simulink model "SVF_fromWorkspace"  (R2018b)
settings: Solver=VariableStepAuto  StartTime=0.0  StopTime=40  RelTol=1e-3
values from neighbouring files (symbols this model uses):
  a0 = omega_n^3    (= 31006276.6803)    [Tflex_Controller_init.m]
  a1 = 3*omega_n^2    (= 296088.132033)    [Tflex_Controller_init.m]
  a2 = 3*omega_n    (= 942.477796077)    [Tflex_Controller_init.m]
  svf_delay = round(svf_delay/(ts*10))    [Tflex_Controller_init.m]
  ts = 1/1000    (= 0.001)    [Tflex_Controller_init.m]
undefined symbols (not defined in the file or in its folder): DiscIntNeverNeededParam
settings Model: Creator=wout7  LastModifiedBy=wout7

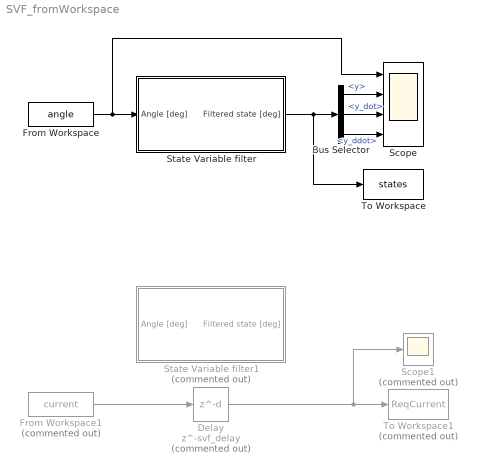
== system SVF_fromWorkspace ==
  Bus Selector : BusSelector  OutputSignals=y,y_dot,y_ddot
  Delay : Delay  Commented=on  DelayLength=svf_delay  SampleTime=ts
  From Workspace : FromWorkspace  VariableName=angle  SampleTime=ts
  From Workspace1 : FromWorkspace  Commented=on  VariableName=current  SampleTime=ts
  Scope : Scope  NumInputPorts=4
  Scope1 : Scope  Commented=on
  State Variable filter : Subsystem
  State Variable filter1 : Subsystem  Commented=on
  To Workspace : ToWorkspace  VariableName=states  SaveFormat=Timeseries  SampleTime=ts
  To Workspace1 : ToWorkspace  Commented=on  VariableName=ReqCurrent  SaveFormat=Timeseries  SampleTime=ts
  wires:
  From Workspace/1 -> Scope/1, State Variable filter/1(Angle [deg])
  State Variable filter/1(Filtered state [deg]) -> To Workspace/1, Bus Selector/1
  Bus Selector/2 -> Scope/3  "<y_dot>"
  Bus Selector/1 -> Scope/2  "<y>"
  Bus Selector/3 -> Scope/4  "<y_ddot>"
  From Workspace1/1 -> Delay/1
  Delay/1 -> Scope1/1, To Workspace1/1

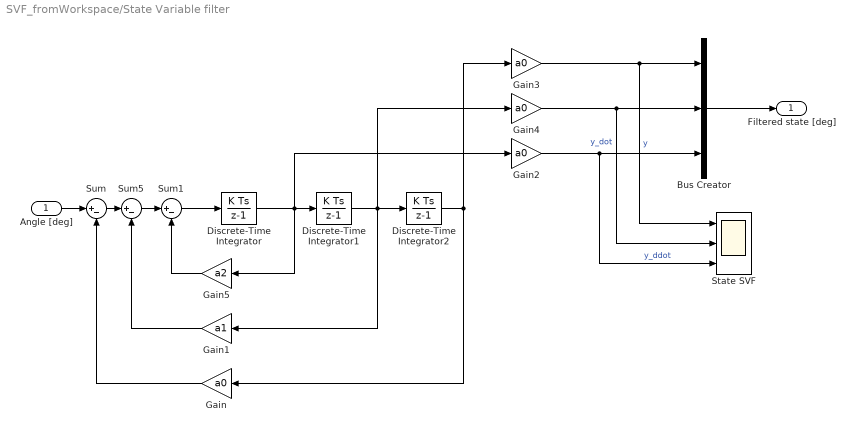
== system SVF_fromWorkspace/State Variable filter ==
  Angle [deg] : Inport
  Bus Creator : BusCreator  Inputs=3
  Discrete-Time Integrator : DiscreteIntegrator  SampleTime=-1  ICPrevOutput=DiscIntNeverNeededParam  ICPrevScaledInput=DiscIntNeverNeededParam
  Discrete-Time Integrator1 : DiscreteIntegrator  SampleTime=-1  ICPrevOutput=DiscIntNeverNeededParam  ICPrevScaledInput=DiscIntNeverNeededParam
  Discrete-Time Integrator2 : DiscreteIntegrator  SampleTime=-1  ICPrevOutput=DiscIntNeverNeededParam  ICPrevScaledInput=DiscIntNeverNeededParam
  Gain{,2..4} (4 alike) : Gain  Gain=a0
  Gain1 : Gain  Gain=a1
  Gain5 : Gain  Gain=a2
  State SVF : Scope  NumInputPorts=3
  Sum : Sum  Inputs=|+-
  Sum1 : Sum  Inputs=|+-
  Sum5 : Sum  Inputs=|+-
  Filtered state [deg] : Outport  SampleTime=ts
  wires:
  Bus Creator/1 -> Filtered state [deg]/1
  Sum1/1 -> Discrete-Time Integrator/1
  Angle [deg]/1 -> Sum/1
  Sum/1 -> Sum5/1
  Gain/1 -> Sum/2
  Gain1/1 -> Sum5/2
  Gain3/1 -> State SVF/1, Bus Creator/1  "y"
  Gain2/1 -> State SVF/3, Bus Creator/3  "y_ddot"
  Gain4/1 -> State SVF/2, Bus Creator/2  "y_dot"
  Gain5/1 -> Sum1/2
  Sum5/1 -> Sum1/1
  Discrete-Time Integrator/1 -> Discrete-Time Integrator1/1, Gain2/1, Gain5/1
  Discrete-Time Integrator1/1 -> Discrete-Time Integrator2/1, Gain4/1, Gain1/1
  Discrete-Time Integrator2/1 -> Gain3/1, Gain/1

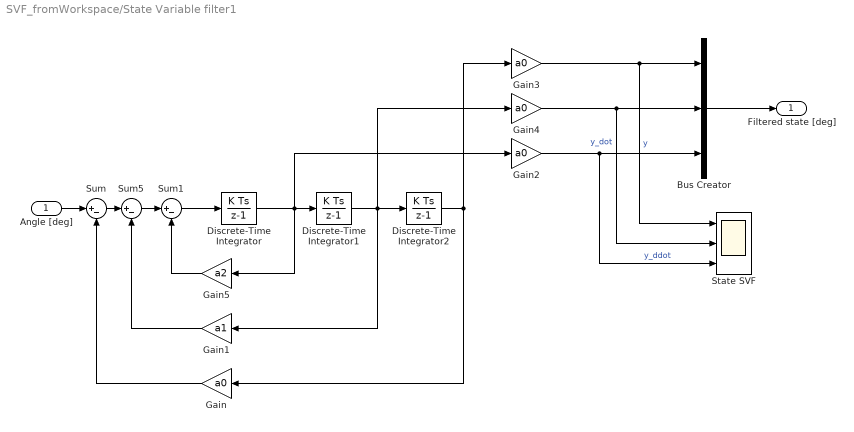
== system SVF_fromWorkspace/State Variable filter1 ==
  Angle [deg] : Inport
  Bus Creator : BusCreator  Inputs=3
  Discrete-Time Integrator : DiscreteIntegrator  SampleTime=-1  ICPrevOutput=DiscIntNeverNeededParam  ICPrevScaledInput=DiscIntNeverNeededParam
  Discrete-Time Integrator1 : DiscreteIntegrator  SampleTime=-1  ICPrevOutput=DiscIntNeverNeededParam  ICPrevScaledInput=DiscIntNeverNeededParam
  Discrete-Time Integrator2 : DiscreteIntegrator  SampleTime=-1  ICPrevOutput=DiscIntNeverNeededParam  ICPrevScaledInput=DiscIntNeverNeededParam
  Gain{,2..4} (4 alike) : Gain  Gain=a0
  Gain1 : Gain  Gain=a1
  Gain5 : Gain  Gain=a2
  State SVF : Scope  NumInputPorts=3
  Sum : Sum  Inputs=|+-
  Sum1 : Sum  Inputs=|+-
  Sum5 : Sum  Inputs=|+-
  Filtered state [deg] : Outport  SampleTime=ts
  wires:
  Bus Creator/1 -> Filtered state [deg]/1
  Sum1/1 -> Discrete-Time Integrator/1
  Angle [deg]/1 -> Sum/1
  Sum/1 -> Sum5/1
  Gain/1 -> Sum/2
  Gain1/1 -> Sum5/2
  Gain3/1 -> State SVF/1, Bus Creator/1  "y"
  Gain2/1 -> State SVF/3, Bus Creator/3  "y_ddot"
  Gain4/1 -> State SVF/2, Bus Creator/2  "y_dot"
  Gain5/1 -> Sum1/2
  Sum5/1 -> Sum1/1
  Discrete-Time Integrator/1 -> Discrete-Time Integrator1/1, Gain2/1, Gain5/1
  Discrete-Time Integrator1/1 -> Discrete-Time Integrator2/1, Gain4/1, Gain1/1
  Discrete-Time Integrator2/1 -> Gain3/1, Gain/1
